simulink model "model2"  (R2021b)
settings: Solver=VariableStepAuto  StartTime=0.0  StopTime=10.0  RelTol=1e-3
values from neighbouring files (symbols this model uses):
  A = [   0    1 ... (first row only)    [config.m]    (also in task2.m = A + [0   0; task3.m = A + [0   0)
  A_m = [     0      1 ... (first row only)    [config.m]
  b = [0 ... (first row only)    [config.m]
  b_m = [0 ... (first row only)    [config.m]
  C = [1 0]    [config.m]
  C_m = C    [config.m]
  kappa = b_0/a_m_0    (= 0.04)    [config.m]
  theta = [theta_1 ... (first row only)    [config.m]
settings Model: Creator=popov  LastModifiedBy=popov

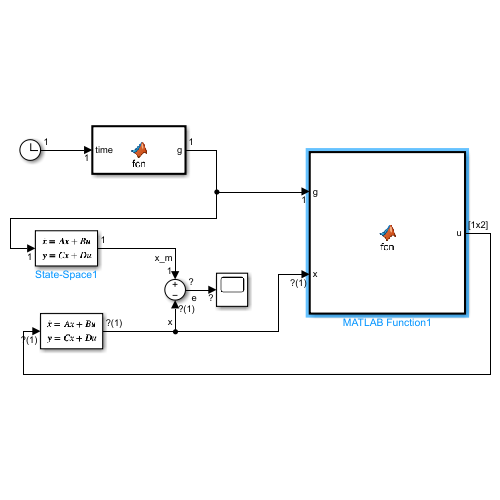
[thumbnail: Simulink's stored preview of the top-level diagram]
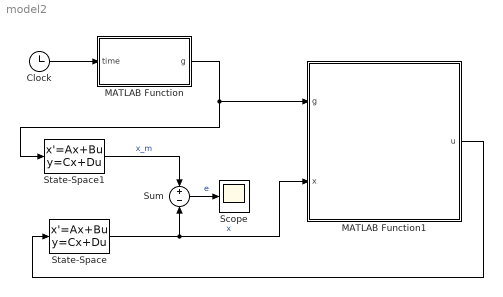
== system model2 ==
  Clock : Clock
  MATLAB Function : MATLAB Function  TreatAsAtomicUnit=on
  MATLAB Function1 : MATLAB Function  TreatAsAtomicUnit=on
  Scope : Scope
  State-Space : StateSpace  A=A  B=b  C=C  D=0  InitialCondition=0
  State-Space1 : StateSpace  A=A_m  B=b_m  C=C_m  D=0  InitialCondition=0
  Sum : Sum  Inputs=+-
  wires:
  Clock/1 -> MATLAB Function/1(time)
  State-Space/1 -> Sum/2, MATLAB Function1/2(x)  "x"
  State-Space1/1 -> Sum/1  "x_m"
  MATLAB Function/1(g) -> State-Space1/1, MATLAB Function1/1(g)
  MATLAB Function1/1(u) -> State-Space/1
  Sum/1 -> Scope/1  "e"

== matlab function model2/MATLAB Function1 ==
  data: g input; x input; u output; kappa parameter; theta parameter
function u  = fcn(g, x, kappa, theta)

u = (theta'*x)+(g/kappa);

== matlab function model2/MATLAB Function ==
  data: time input; g output
function g = fcn(time)

g = 2*sign(sin(0.4*time)) + 3;
